simulink model "chinese_missile_block_diagrams"  (R2023b)
settings: Solver=VariableStepAuto  StartTime=0.0  StopTime=10.0  RelTol=1e-3
values from neighbouring files (symbols this model uses):
  resol = 1000    [ispitany.m]    (also in missile_data_analyzer.m)
libraries: slpidlib x2
settings Model: Creator=n8dsa  LastModifiedBy=n8dsa

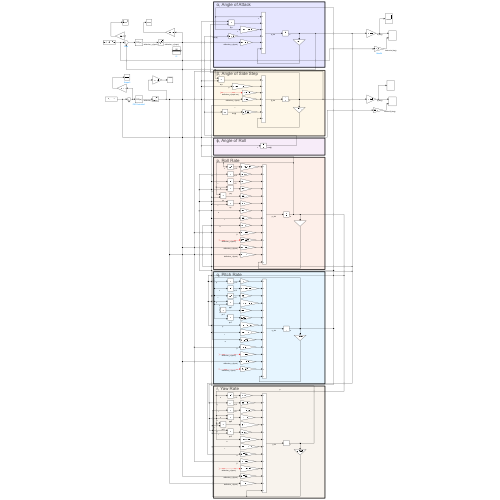
[thumbnail: Simulink's stored preview of the top-level diagram]
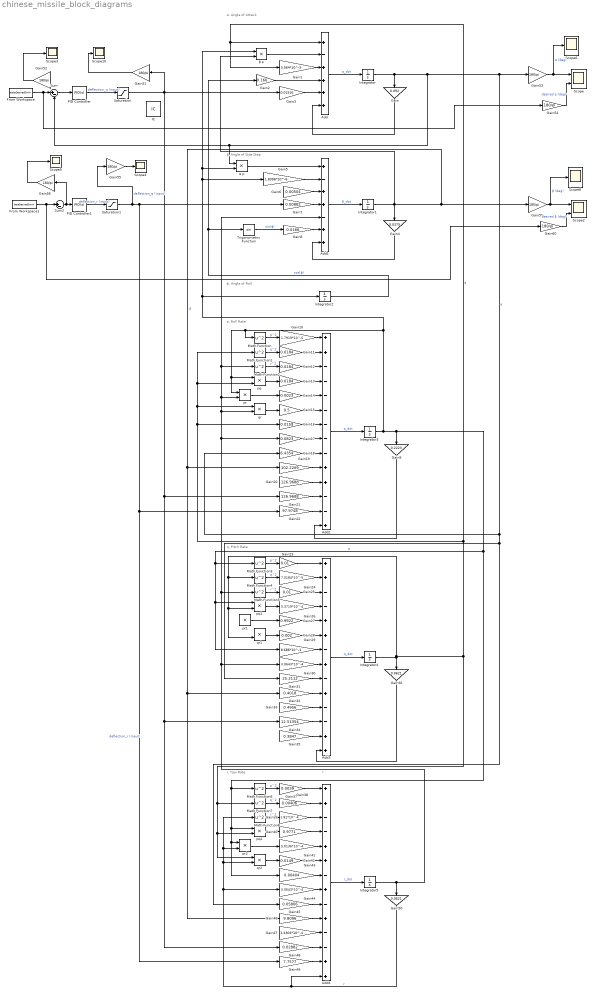
== system chinese_missile_block_diagrams ==
  note: α, Angle of Attack
  note: β, Angle of Side Step
  note: ɸ, Angle of Roll
  note: p, Roll Rate
  note: q, Pitch Rate
  note: r, Yaw Rate
  Add : Sum  Inputs=+-++++
  Add1 : Sum  Inputs=+-++-++
  Add2 : Sum  Inputs=++-------++--+
  Add3 : Sum  Inputs=++--++-+-+--++
  Add4 : Sum  Inputs=++--++-+-+--++
  From Workspace : FromWorkspace  VariableName=alphaDesiredSimIn  SampleTime=1/resol
  From Workspace1 : FromWorkspace  VariableName=betaDesiredSimIn  SampleTime=1/resol
  Gain : Gain  Gain=0.092
  Gain1 : Gain  Gain=3.564*10^-5
  Gain10 : Gain  Gain=1.7919*10^-5
  Gain11 : Gain  Gain=0.0184
  Gain12 : Gain  Gain=0.0184
  Gain13 : Gain  Gain=0.0184
  Gain14 : Gain  Gain=0.0023
  Gain15 : Gain  Gain=0.5
  Gain16 : Gain  Gain=0.0159
  Gain17 : Gain  Gain=0.0823
  Gain18 : Gain  Gain=6.4354
  Gain19 : Gain  Gain=102.2269
  Gain2 : Gain  Gain=0.166
  Gain20 : Gain  Gain=126.9688
  Gain21 : Gain  Gain=126.9688
  Gain22 : Gain  Gain=97.9748
  Gain23 : Gain  Gain=0.01
  Gain24 : Gain  Gain=7.0184*10^-5
  Gain25 : Gain  Gain=0.01
  Gain26 : Gain  Gain=5.3719*10^-4
  Gain27 : Gain  Gain=0.9922
  Gain28 : Gain  Gain=0.002
  Gain29 : Gain  Gain=8.686*10^-4
  Gain3 : Gain  Gain=0.01516
  Gain30 : Gain  Gain=3.0643*10^-4
  Gain31 : Gain  Gain=25.2112
  Gain32 : Gain  Gain=0.4018
  Gain33 : Gain  Gain=0.4956
  Gain34 : Gain  Gain=12.51354
  Gain35 : Gain  Gain=0.3847
  Gain36 : Gain  Gain=0.0621
  Gain37 : Gain  Gain=0.0039
  Gain38 : Gain  Gain=0.00406
  Gain39 : Gain  Gain=1.81*10^-4
  Gain4 : Gain  Gain=0.0375
  Gain40 : Gain  Gain=0.9771
  Gain41 : Gain  Gain=5.0136*10^-4
  Gain42 : Gain  Gain=0.0149
  Gain43 : Gain  Gain=0.00404
  Gain44 : Gain  Gain=3.0643*10^-4
  Gain45 : Gain  Gain=0.05806
  Gain46 : Gain  Gain=9.8096
  Gain47 : Gain  Gain=1.4304*10^-4
  Gain48 : Gain  Gain=0.02882
  Gain49 : Gain  Gain=7.7577
  Gain5 : Gain  Gain=1.8396*10^-6
  Gain50 : Gain  Gain=0.0621
  Gain{51..56,59..60} (8 alike) : Gain  Gain=180/pi
  Gain6 : Gain  Gain=0.00504
  Gain7 : Gain  Gain=0.00882
  Gain8 : Gain  Gain=0.0166
  Gain9 : Gain  Gain=0.2223
  IC : InitialCondition  Value=0
  Integrator{,1..5} (6 alike) : Integrator
  Math Function{,1..8} (9 alike) : Math  Operator=square
  PID Controller : slpidlib/PID Controller  Controller=PID  Form=Parallel  TimeDomain=Continuous-time  UseExternalTs=off  SampleTime=-1  IntegratorMethod=Forward Euler  FilterMethod=Forward Euler  ControllerParametersSource=internal  P=-22.41452785697  I=-44.4417011508284  UseKiTs=off  D=-2.7314154579227  N=377.085826848112  UseFilter=on  TunerSelectOption=Transfer Function Based (PID Tuner App)  InitialConditionSource=internal  InitialConditionForIntegrator=0  InitialConditionForFilter=0  DifferentiatorICPrevScaledInput=0  ExternalReset=none  TrackingMode=off  Kt=1  LimitOutput=off  SatLimitsSource=internal  UpperSaturationLimit=inf  LowerSaturationLimit=-inf  LinearizeAsGain=on  AntiWindupMode=none  Kb=1  LimitIntegrator=off  UpperIntegratorSaturationLimit=inf  LowerIntegratorSaturationLimit=-inf  POutMin=[]  POutMax=[]  IOutMin=[]  IOutMax=[]  DOutMin=[]  DOutMax=[]  NOutMin=[]  NOutMax=[]  SumOutMin=[]  SumOutMax=[]  SaturationOutMin=[]  SaturationOutMax=[]  PParamMin=[]  PParamMax=[]  IParamMin=[]  IParamMax=[]  DParamMin=[]  DParamMax=[]  NParamMin=[]  NParamMax=[]  KbParamMin=[]  KbParamMax=[]  KtParamMin=[]  KtParamMax=[]  KbOutMin=[]  KbOutMax=[]  KtOutMin=[]  KtOutMax=[]  IntegratorOutMin=[]  IntegratorOutMax=[]  FilterOutMin=[]  FilterOutMax=[]  SumI1OutMin=[]  SumI1OutMax=[]  SumI2OutMin=[]  SumI2OutMax=[]  SumI3OutMin=[]  SumI3OutMax=[]  SumI4OutMin=[]  SumI4OutMax=[]  SumDOutMin=[]  SumDOutMax=[]  DifferentiatorOutMin=[]  DifferentiatorOutMax=[]  FilterDiffOutCoefMin=[]  FilterDiffOutCoefMax=[]  ReciprocalOutMin=[]  ReciprocalOutMax=[]  SumDenOutMin=[]  SumDenOutMax=[]  SumNumOutMin=[]  SumNumOutMax=[]  DivideOutMin=[]  DivideOutMax=[]  UdiffTsProdOutMin=[]  UdiffTsProdOutMax=[]  NTsProdOutMin=[]  NTsProdOutMax=[]  UintegralTsProdOutMin=[]  UintegralTsProdOutMax=[]  UngainTsProdOutMin=[]  UngainTsProdOutMax=[]  ClampingZeroOutDataTypeStr=Inherit: Inherit via back propagation  ClampingZeroOutMin=[]  ClampingZeroOutMax=[]  FilterDenConstantOutDataTypeStr=Inherit: Inherit via back propagation  FilterDenConstantOutMin=[]  FilterDenConstantOutMax=[]  PCopyOutDataTypeStr=Inherit: Inherit via back propagation  PCopyOutMin=[]  PCopyOutMax=[]  NCopyOutDataTypeStr=Inherit: Inherit via back propagation  NCopyOutMin=[]  NCopyOutMax=[]  IntegratorContinuousStateAttributes=''  IntegratorStateMustResolveToSignalObject=off  IntegratorRTWStateStorageClass=Auto  FilterContinuousStateAttributes=''  FilterStateMustResolveToSignalObject=off  FilterRTWStateStorageClass=Auto  ParallelPVariant=InternalParameters  IdealPVariant=Disabled  IVariant=InternalParameters  DVariant=InternalParameters  IntegratorVariant=Continuous  SatVariant=Disabled  AWVariant=Passthrough  PCopyVariant=Disabled  TRVariant=Disabled  FdbkBlocksVariant=Forward  IdealPFdbkVariant=Disabled  SatFdbkVariant=Disabled  DerivativeFilterVariant=ContFilter  NVariant=InternalParameters  NCopyVariant=Disabled  FilterICVariant=InternalICsFilter  IntegratorICVariant=InternalICs  ExternalResetVariant=Disabled  TRSumVariant=Passthrough  SumFdbkVariant=Disabled  SumVariant=Sum_PID  TsampFilterVariant=InternalTs  TsampNgainVariant=Passthrough  TsampIntegralVariant=Disabled_SignalSpec  ExternalSaturationOutDataTypeStr=Inherit: Same as second input
  PID Controller1 : slpidlib/PID Controller  Controller=PID  Form=Parallel  TimeDomain=Continuous-time  UseExternalTs=off  SampleTime=-1  IntegratorMethod=Forward Euler  FilterMethod=Forward Euler  ControllerParametersSource=internal  P=-12.6163733675251  I=-15.0679855193864  UseKiTs=off  D=-2.48145523449249  N=214.117607967153  UseFilter=on  TunerSelectOption=Transfer Function Based (PID Tuner App)  InitialConditionSource=internal  InitialConditionForIntegrator=0  InitialConditionForFilter=0  DifferentiatorICPrevScaledInput=0  ExternalReset=none  TrackingMode=off  Kt=1  LimitOutput=off  SatLimitsSource=internal  UpperSaturationLimit=inf  LowerSaturationLimit=-inf  LinearizeAsGain=on  AntiWindupMode=none  Kb=1  LimitIntegrator=off  UpperIntegratorSaturationLimit=inf  LowerIntegratorSaturationLimit=-inf  POutMin=[]  POutMax=[]  IOutMin=[]  IOutMax=[]  DOutMin=[]  DOutMax=[]  NOutMin=[]  NOutMax=[]  SumOutMin=[]  SumOutMax=[]  SaturationOutMin=[]  SaturationOutMax=[]  PParamMin=[]  PParamMax=[]  IParamMin=[]  IParamMax=[]  DParamMin=[]  DParamMax=[]  NParamMin=[]  NParamMax=[]  KbParamMin=[]  KbParamMax=[]  KtParamMin=[]  KtParamMax=[]  KbOutMin=[]  KbOutMax=[]  KtOutMin=[]  KtOutMax=[]  IntegratorOutMin=[]  IntegratorOutMax=[]  FilterOutMin=[]  FilterOutMax=[]  SumI1OutMin=[]  SumI1OutMax=[]  SumI2OutMin=[]  SumI2OutMax=[]  SumI3OutMin=[]  SumI3OutMax=[]  SumI4OutMin=[]  SumI4OutMax=[]  SumDOutMin=[]  SumDOutMax=[]  DifferentiatorOutMin=[]  DifferentiatorOutMax=[]  FilterDiffOutCoefMin=[]  FilterDiffOutCoefMax=[]  ReciprocalOutMin=[]  ReciprocalOutMax=[]  SumDenOutMin=[]  SumDenOutMax=[]  SumNumOutMin=[]  SumNumOutMax=[]  DivideOutMin=[]  DivideOutMax=[]  UdiffTsProdOutMin=[]  UdiffTsProdOutMax=[]  NTsProdOutMin=[]  NTsProdOutMax=[]  UintegralTsProdOutMin=[]  UintegralTsProdOutMax=[]  UngainTsProdOutMin=[]  UngainTsProdOutMax=[]  ClampingZeroOutDataTypeStr=Inherit: Inherit via back propagation  ClampingZeroOutMin=[]  ClampingZeroOutMax=[]  FilterDenConstantOutDataTypeStr=Inherit: Inherit via back propagation  FilterDenConstantOutMin=[]  FilterDenConstantOutMax=[]  PCopyOutDataTypeStr=Inherit: Inherit via back propagation  PCopyOutMin=[]  PCopyOutMax=[]  NCopyOutDataTypeStr=Inherit: Inherit via back propagation  NCopyOutMin=[]  NCopyOutMax=[]  IntegratorContinuousStateAttributes=''  IntegratorStateMustResolveToSignalObject=off  IntegratorRTWStateStorageClass=Auto  FilterContinuousStateAttributes=''  FilterStateMustResolveToSignalObject=off  FilterRTWStateStorageClass=Auto  ParallelPVariant=InternalParameters  IdealPVariant=Disabled  IVariant=InternalParameters  DVariant=InternalParameters  IntegratorVariant=Continuous  SatVariant=Disabled  AWVariant=Passthrough  PCopyVariant=Disabled  TRVariant=Disabled  FdbkBlocksVariant=Forward  IdealPFdbkVariant=Disabled  SatFdbkVariant=Disabled  DerivativeFilterVariant=ContFilter  NVariant=InternalParameters  NCopyVariant=Disabled  FilterICVariant=InternalICsFilter  IntegratorICVariant=InternalICs  ExternalResetVariant=Disabled  TRSumVariant=Passthrough  SumFdbkVariant=Disabled  SumVariant=Sum_PID  TsampFilterVariant=InternalTs  TsampNgainVariant=Passthrough  TsampIntegralVariant=Disabled_SignalSpec  ExternalSaturationOutDataTypeStr=Inherit: Same as second input
  Saturation : Saturate  UpperLimit=pi*50/180  LowerLimit=-pi*50/180
  Saturation1 : Saturate  UpperLimit=pi*50/180  LowerLimit=-pi*50/180
  Scope : Scope  NumInputPorts=2
  Scope{3..6,8,10} (6 alike) : Scope
  Scope2 : Scope  NumInputPorts=2
  Sum : Sum  Inputs=|+-
  Sum2 : Sum  Inputs=|+-
  Trigonometric Function : Trigonometry
  pq : Product
  pq1 : Product
  pq2 : Product
  pr : Product
  pr1 : Product
  pr2 : Product
  qr : Product
  qr1 : Product
  qr2 : Product
  α p : Product
  β p : Product
  wires:
  Add/1 -> Integrator/1  "α_dot"
  Gain/1 -> Add/6
  β p/1 -> Add/2
  Gain1/1 -> Add/3
  Integrator4/1 -> Gain1/1, Add/1, pq/2, Math Function1/1, qr/1, Gain16/1, qr2/1, pq2/2, Math Function7/1, qr1/2, pq1/2, Math Function4/1, Gain36/1  "q"
  Gain2/1 -> Add/4
  Integrator2/1 -> Gain2/1, Trigonometric Function/1  "cos(ɸ)"
  Gain3/1 -> Add/5
  Add1/1 -> Integrator1/1  "β_dot"
  Gain4/1 -> Add1/7
  α p/1 -> Add1/1
  Gain5/1 -> Add1/2
  Integrator3/1 -> pq/1, pr/1, Math Function/1, β p/1, α p/2, Gain5/1, Integrator2/1, pq1/1, Gain29/1, Math Function3/1, pq2/1, Gain43/1, pr2/1, Math Function6/1, Gain9/1  "p"
  Gain6/1 -> Add1/3
  ? -> Gain6/1  "deflection_p (input var)"
  Gain7/1 -> Add1/4
  Integrator5/1 -> Gain30/1, Math Function5/1, Add1/5, Math Function2/1, pr/2, qr/2, Gain17/1, Gain50/1  "r"
  Gain8/1 -> Add1/6
  Trigonometric Function/1 -> Gain8/1  "sin(ɸ)"
  Add2/1 -> Integrator3/1  "p_dot"
  Math Function/1 -> Gain10/1  "p^2"
  Gain10/1 -> Add2/1
  Math Function1/1 -> Gain11/1  "q^2"
  Gain11/1 -> Add2/2
  Math Function2/1 -> Gain12/1  "r^2"
  Gain12/1 -> Add2/3
  pq/1 -> Gain13/1
  Gain13/1 -> Add2/4
  Gain14/1 -> Add2/5
  pr/1 -> Gain14/1
  Gain15/1 -> Add2/6
  qr/1 -> Gain15/1
  Gain9/1 -> Add2/14
  Gain16/1 -> Add2/7
  Gain17/1 -> Add2/8
  Gain18/1 -> Add2/9
  Gain19/1 -> Add2/10
  Gain20/1 -> Add2/11
  ? -> Gain20/1  "deflection_p (input)"
  Gain21/1 -> Add2/12
  Saturation/1 -> Gain21/1, Gain34/1, Gain48/1, Gain51/1, Gain3/1  "deflection_q (input)"
  Gain22/1 -> Add2/13
  Saturation1/1 -> Gain22/1, Gain49/1, Gain7/1, Gain55/1  "deflection_r (input)"
  ? -> Gain35/1  "deflection_r (input)"
  ? -> Gain33/1  "deflection_p (input)"
  Integrator1/1 -> β p/2, Gain59/1, Gain19/1, Gain32/1, Gain46/1, Gain4/1  "β"
  Integrator/1 -> Gain31/1, Gain45/1, Gain18/1, Gain53/1, Sum/2, α p/1, Gain/1  "α"
  Math Function4/1 -> Gain24/1  "q^2"
  Gain36/1 -> Add3/14
  Gain34/1 -> Add3/12
  Gain30/1 -> Add3/8
  Gain33/1 -> Add3/11
  Gain26/1 -> Add3/4
  Gain28/1 -> Add3/6
  pq1/1 -> Gain26/1
  Gain27/1 -> Add3/5
  Gain29/1 -> Add3/7
  pr1/1 -> Gain27/1
  Math Function3/1 -> Gain23/1  "p^2"
  qr1/1 -> Gain28/1
  Gain24/1 -> Add3/2
  Gain31/1 -> Add3/9
  Gain23/1 -> Add3/1
  Gain35/1 -> Add3/13
  Add3/1 -> Integrator4/1  "q_dot"
  Gain25/1 -> Add3/3
  Math Function5/1 -> Gain25/1  "r^2"
  Gain32/1 -> Add3/10
  Gain46/1 -> Add4/10
  Gain48/1 -> Add4/12
  Math Function7/1 -> Gain38/1  "q^2"
  Gain50/1 -> Gain44/1, qr2/2, pr2/2, Math Function8/1, Add4/14  "r"
  ? -> Gain47/1  "deflection_p (input)"
  Gain47/1 -> Add4/11
  Gain43/1 -> Add4/7
  Gain42/1 -> Add4/6
  Math Function6/1 -> Gain37/1  "p^2"
  Gain41/1 -> Add4/5
  pr2/1 -> Gain41/1
  pq2/1 -> Gain40/1
  Gain44/1 -> Add4/8
  Math Function8/1 -> Gain39/1  "r^2"
  Gain39/1 -> Add4/3
  Gain49/1 -> Add4/13
  Gain40/1 -> Add4/4
  Add4/1 -> Integrator5/1  "r_dot"
  Gain37/1 -> Add4/1
  Gain45/1 -> Add4/9
  qr2/1 -> Gain42/1
  Gain38/1 -> Add4/2
  Sum/1 -> PID Controller/1
  From Workspace/1 -> Gain54/1, Sum/1
  Gain52/1 -> Scope3/1
  PID Controller/1 -> Saturation/1  "deflection_q (input)"
  Gain51/1 -> Scope10/1
  Gain53/1 -> Scope6/1, Scope/1  "α (deg)"
  Gain54/1 -> Scope/2  "desired α (deg)"
  From Workspace1/1 -> Gain60/1, Sum2/1
  Sum2/1 -> Gain56/1, PID Controller1/1
  PID Controller1/1 -> Saturation1/1  "deflection_r (input)"
  Gain56/1 -> Scope5/1
  Gain55/1 -> Scope4/1
  Gain60/1 -> Scope2/2  "desired β (deg)"
  Gain59/1 -> Scope8/1, Scope2/1  "β (deg)"
